simulink model "Biped_Model"  (R2019a)
settings: Solver=VariableStepAuto  StartTime=0.0  StopTime=Time(end)  FixedStep=.001  EnableMultiTasking=on
PreLoadFcn:
  | YBT_HomeDir = pwd;
  | 
  | % Code to use copy within this repository
  | addpath([YBT_HomeDir filesep 'Libraries' filesep 'CFL_Libs']);
  | startup_Contact_Forces
  | 
  | cd(YBT_HomeDir)
  | addpath(YBT_HomeDir);
  | addpath([YBT_HomeDir filesep 'Libraries']);
  | addpath([YBT_HomeDir filesep 'Images']);
  | 
  | Robot_Parameters
model workspace: external: MATLAB File C:\Users\nozaripo\Desktop\BipedalWalking_Simulink_ModelnData\Robot_Parameters.m (data not in the file)
values from neighbouring files (symbols this model uses):
  ankle_servo_kd = 4    [Robot_Parameters.m]
  ankle_servo_ki = 0    [Robot_Parameters.m]
  ankle_servo_kp = 70    [Robot_Parameters.m]
  ankle_to_midLow = 19    [Robot_Parameters.m]
  contact_damping = 50    [Robot_Parameters.m]
  contact_point_radius = 0.005    [Robot_Parameters.m]
  contact_stiffness = 90311    [Robot_Parameters.m]
  deriv_filter_coeff = 50    [Robot_Parameters.m]
  foot_mass = 1    [Robot_Parameters.m]
  height_plane = 0.1    [Robot_Parameters.m]
  hip_servo_kd = 30    [Robot_Parameters.m]
  hip_servo_ki = 0    [Robot_Parameters.m]
  hip_servo_kp = 300    [Robot_Parameters.m]
  init = -joint_angles(1,:)    [Script_Data.m]
  init_vel = -vel(1,:)    [Script_Data.m]
  joint_angles = joint_angles(:,end:-1:1)    [Script_Data.m]
  joint_damping = 0    [Robot_Parameters.m]
  joint_stiffness = 0    [Robot_Parameters.m]
  knee_servo_kd = 30    [Robot_Parameters.m]
  knee_servo_ki = 0    [Robot_Parameters.m]
  knee_servo_kp = 150    [Robot_Parameters.m]
  knee_to_midUpp = 19    [Robot_Parameters.m]
  linear_contact_flag = 0    [Robot_Parameters.m]
  lower_leg_CM_offset = 2.55    [Robot_Parameters.m]
  lower_leg_mass = 2.87    [Robot_Parameters.m]
  max_torque_ank = 45    [Robot_Parameters.m]
  max_torque_hip = 25    [Robot_Parameters.m]
  max_torque_kn = 30    [Robot_Parameters.m]
  midLow_to_knee = 19    [Robot_Parameters.m]
  midUpp_to_hip = 19    [Robot_Parameters.m]
  motion_time_constant = 0.01    [Robot_Parameters.m]
  motor_constant = 0.01    [Robot_Parameters.m]
  motor_inertia = 0    [Robot_Parameters.m]
  mu_k = 0.5    [Robot_Parameters.m]
  mu_s = 0.8    [Robot_Parameters.m]
  mu_vth = 0.1    [Robot_Parameters.m]
  pen_exp = 1.5    [Robot_Parameters.m]
  plane_x = 3    [Robot_Parameters.m]
  plane_y = 0.3    [Robot_Parameters.m]
  split_belt = 0    [Script_Data.m]
  Time = (0:.01:.01*209)'    [Script_Data.m]
  torso_mass = 27.17    [Robot_Parameters.m]
  torso_to_hip = 11    [Robot_Parameters.m]
  upper_leg_CM_offset = 2.55    [Robot_Parameters.m]
  upper_leg_length = 38    [Robot_Parameters.m]
  upper_leg_mass = 4.7    [Robot_Parameters.m]
  V_treadmill = -1.0    (= -1)    [Script_Data.m]
  YBT_Par = struct    [Robot_Parameters.m]
undefined symbols (not defined in the file or in its folder): Extr_Data_LinkHoles, X, Y, Z
libraries: nesl_utility x198, sm_lib x144, fl_lib x42, simulink x20, ee_lib x18, Contact_Forces_Lib x16, Parts_Lib x10, Multibody_Multiphysics_Lib x6, simulink_extras x1
(part 9 of 11)

== system Biped_Model/Robot/Robot Leg R/Package Measurements/Extract Measurements1 ==
  meas : Inport
  Bus Selector : BusSelector  OutputSignals=angle,speed,torque
  angle : Outport
  speed : Outport  Port=2
  torque : Outport  Port=3
  wires:
  Bus Selector/3 -> torque/1  "<torque>"
  meas/1 -> Bus Selector/1
  Bus Selector/1 -> angle/1  "<angle>"
  Bus Selector/2 -> speed/1  "<speed>"

== system Biped_Model/Robot/Robot Leg R/Package Measurements/Extract Measurements2 ==
  meas : Inport
  Bus Selector : BusSelector  OutputSignals=angle,speed,torque
  angle : Outport
  speed : Outport  Port=2
  torque : Outport  Port=3
  wires:
  Bus Selector/1 -> angle/1  "<angle>"
  meas/1 -> Bus Selector/1
  Bus Selector/3 -> torque/1  "<torque>"
  Bus Selector/2 -> speed/1  "<speed>"

== system Biped_Model/Robot/Robot Leg L/Ankle Joint/Motor/Joint Servo ==
  qref : Inport
  Abs : Abs
  Controlled Voltage Source : fl_lib/Electrical/Electrical Sources/Controlled Voltage Source
  Controlled Voltage Source1 : fl_lib/Electrical/Electrical Sources/Controlled Voltage Source
  Electrical Reference : fl_lib/Electrical/Electrical Elements/Electrical Reference
  PID Controller : simulink/Continuous/PID Controller  Controller=PID  Form=Parallel  TimeDomain=Continuous-time  SampleTime=-1  IntegratorMethod=Forward Euler  FilterMethod=Forward Euler  ControllerParametersSource=internal  P=Kp  I=Ki  D=Kd  UseFilter=on  N=N  TunerSelectOption=Transfer Function Based (PID Tuner App)  ZeroCross=off  InitialConditionSource=internal  InitialConditionForIntegrator=0  InitialConditionForFilter=0  DifferentiatorICPrevScaledInput=0  ExternalReset=none  TrackingMode=off  Kt=1  LimitOutput=on  UpperSaturationLimit=Tmax  LowerSaturationLimit=-Tmax  LinearizeAsGain=on  AntiWindupMode=clamping  Kb=1  POutMin=[]  POutMax=[]  IOutMin=[]  IOutMax=[]  DOutMin=[]  DOutMax=[]  NOutMin=[]  NOutMax=[]  SumOutMin=[]  SumOutMax=[]  SaturationOutMin=[]  SaturationOutMax=[]  PParamMin=[]  PParamMax=[]  IParamMin=[]  IParamMax=[]  DParamMin=[]  DParamMax=[]  NParamMin=[]  NParamMax=[]  KbParamMin=[]  KbParamMax=[]  KtParamMin=[]  KtParamMax=[]  KbOutMin=[]  KbOutMax=[]  KtOutMin=[]  KtOutMax=[]  IntegratorOutMin=[]  IntegratorOutMax=[]  FilterOutMin=[]  FilterOutMax=[]  SumI1OutMin=[]  SumI1OutMax=[]  SumI2OutMin=[]  SumI2OutMax=[]  SumI3OutMin=[]  SumI3OutMax=[]  SumI4OutMin=[]  SumI4OutMax=[]  SumDOutMin=[]  SumDOutMax=[]  DifferentiatorOutMin=[]  DifferentiatorOutMax=[]  FilterDiffOutCoefMin=[]  FilterDiffOutCoefMax=[]  ReciprocalOutMin=[]  ReciprocalOutMax=[]  SumDenOutMin=[]  SumDenOutMax=[]  SumNumOutMin=[]  SumNumOutMax=[]  DivideOutMin=[]  DivideOutMax=[]  IntegratorContinuousStateAttributes=''  IntegratorStateMustResolveToSignalObject=off  IntegratorRTWStateStorageClass=Auto  FilterContinuousStateAttributes=''  FilterStateMustResolveToSignalObject=off  FilterRTWStateStorageClass=Auto  ParallelPVariant=InternalParameters  IdealPVariant=Disabled  IVariant=InternalParameters  DVariant=InternalParameters  IntegratorVariant=Continuous  SatVariant=Enabled  AWVariant=ContClampingParallel  PCopyVariant=Disabled  TRVariant=Disabled  FdbkBlocksVariant=Forward  IdealPFdbkVariant=Disabled  SatFdbkVariant=Disabled  DerivativeFilterVariant=ContFilter  NVariant=InternalParameters  NCopyVariant=Disabled  FilterICVariant=InternalICsFilter  IntegratorICVariant=InternalICs  ExternalResetVariant=Disabled  TRSumVariant=Passthrough  SumFdbkVariant=Disabled  SumVariant=Sum_PID
  PS-Simulink Converter : nesl_utility/PS-Simulink Converter  PhysicalDomain=network_engine_domain  SubClassName=ps_output  LeftPortType=input  RightPortType=output  PseudoPeriodic=off  Frequencies=[]  Unit=rad  AffineConversion=off
  Relay : Relay  OnSwitchValue=1e-3  OffSwitchValue=-1e-3  OnOutputValue=0  OffOutputValue=5
  Simulink-PS Converter : nesl_utility/Simulink-PS Converter  PhysicalDomain=network_engine_domain  SubClassName=ps_input  LeftPortType=input  RightPortType=output  PseudoPeriodic=off  Frequencies=[]  NoiseDistribution=none  NoiseParameters=[]  Unit=1  AffineConversion=off  FilteringAndDerivatives=provide  SimscapeFilterOrder=1  InputFilterTimeConstant=0.005  UdotUserProvided=0
  Simulink-PS Converter1 : nesl_utility/Simulink-PS Converter  PhysicalDomain=network_engine_domain  SubClassName=ps_input  LeftPortType=input  RightPortType=output  PseudoPeriodic=off  Frequencies=[]  NoiseDistribution=none  NoiseParameters=[]  Unit=1  AffineConversion=off  FilteringAndDerivatives=provide  SimscapeFilterOrder=1  InputFilterTimeConstant=0.005  UdotUserProvided=0
  Sum : Sum  Inputs=|+-
  q : PMIOPort  Side=Left
  V : PMIOPort  Port=2  Side=Right
  REV : PMIOPort  Port=3  Side=Right
  wires:
  PID Controller/1 -> Abs/1, Relay/1
  qref/1 -> Sum/1
  PS-Simulink Converter/1 -> Sum/2
  Sum/1 -> PID Controller/1
  Abs/1 -> Simulink-PS Converter/1
  Relay/1 -> Simulink-PS Converter1/1
  connections:
  q/RConn1 -- PS-Simulink Converter/LConn1
  Simulink-PS Converter/RConn1 -- Controlled Voltage Source/RConn1
  Controlled Voltage Source/LConn1 -- V/RConn1
  Electrical Reference/LConn1 -- Controlled Voltage Source/RConn2 -- Controlled Voltage Source1/RConn2
  Controlled Voltage Source1/LConn1 -- REV/RConn1
  Simulink-PS Converter1/RConn1 -- Controlled Voltage Source1/RConn1

== system Biped_Model/Robot/Robot Leg L/Ankle Joint/Torque/Joint Servo ==
  qref : Inport
  Memory : Memory
  PID Controller : simulink/Continuous/PID Controller  Controller=PID  Form=Parallel  TimeDomain=Continuous-time  SampleTime=-1  IntegratorMethod=Forward Euler  FilterMethod=Forward Euler  ControllerParametersSource=internal  P=Kp  I=Ki  D=Kd  UseFilter=on  N=N  TunerSelectOption=Transfer Function Based (PID Tuner App)  ZeroCross=off  InitialConditionSource=internal  InitialConditionForIntegrator=0  InitialConditionForFilter=0  DifferentiatorICPrevScaledInput=0  ExternalReset=none  TrackingMode=off  Kt=1  LimitOutput=on  UpperSaturationLimit=Tmax  LowerSaturationLimit=-Tmax  LinearizeAsGain=on  AntiWindupMode=clamping  Kb=1  POutMin=[]  POutMax=[]  IOutMin=[]  IOutMax=[]  DOutMin=[]  DOutMax=[]  NOutMin=[]  NOutMax=[]  SumOutMin=[]  SumOutMax=[]  SaturationOutMin=[]  SaturationOutMax=[]  PParamMin=[]  PParamMax=[]  IParamMin=[]  IParamMax=[]  DParamMin=[]  DParamMax=[]  NParamMin=[]  NParamMax=[]  KbParamMin=[]  KbParamMax=[]  KtParamMin=[]  KtParamMax=[]  KbOutMin=[]  KbOutMax=[]  KtOutMin=[]  KtOutMax=[]  IntegratorOutMin=[]  IntegratorOutMax=[]  FilterOutMin=[]  FilterOutMax=[]  SumI1OutMin=[]  SumI1OutMax=[]  SumI2OutMin=[]  SumI2OutMax=[]  SumI3OutMin=[]  SumI3OutMax=[]  SumI4OutMin=[]  SumI4OutMax=[]  SumDOutMin=[]  SumDOutMax=[]  DifferentiatorOutMin=[]  DifferentiatorOutMax=[]  FilterDiffOutCoefMin=[]  FilterDiffOutCoefMax=[]  ReciprocalOutMin=[]  ReciprocalOutMax=[]  SumDenOutMin=[]  SumDenOutMax=[]  SumNumOutMin=[]  SumNumOutMax=[]  DivideOutMin=[]  DivideOutMax=[]  IntegratorContinuousStateAttributes=''  IntegratorStateMustResolveToSignalObject=off  IntegratorRTWStateStorageClass=Auto  FilterContinuousStateAttributes=''  FilterStateMustResolveToSignalObject=off  FilterRTWStateStorageClass=Auto  ParallelPVariant=InternalParameters  IdealPVariant=Disabled  IVariant=InternalParameters  DVariant=InternalParameters  IntegratorVariant=Continuous  SatVariant=Enabled  AWVariant=ContClampingParallel  PCopyVariant=Disabled  TRVariant=Disabled  FdbkBlocksVariant=Forward  IdealPFdbkVariant=Disabled  SatFdbkVariant=Disabled  DerivativeFilterVariant=ContFilter  NVariant=InternalParameters  NCopyVariant=Disabled  FilterICVariant=InternalICsFilter  IntegratorICVariant=InternalICs  ExternalResetVariant=Disabled  TRSumVariant=Passthrough  SumFdbkVariant=Disabled  SumVariant=Sum_PID
  PS-Simulink Converter : nesl_utility/PS-Simulink Converter  PhysicalDomain=network_engine_domain  SubClassName=ps_output  LeftPortType=input  RightPortType=output  PseudoPeriodic=off  Frequencies=[]  Unit=rad  AffineConversion=off
  Sum : Sum  Inputs=|+-
  q : PMIOPort  Side=Left
  t : Outport
  wires:
  PID Controller/1 -> t/1
  Sum/1 -> PID Controller/1
  PS-Simulink Converter/1 -> Memory/1
  qref/1 -> Sum/1
  Memory/1 -> Sum/2
  connections:
  q/RConn1 -- PS-Simulink Converter/LConn1

== system Biped_Model/Robot/Robot Leg L/Box to Belt In Force1/Sphere to Plane Force Enabled nz1/Check Sphere on Plane ==
  x : Inport
  y : Inport  Port=2
  Abs : Abs  ZeroCross=off
  Abs1 : Abs  ZeroCross=off
  Check loc x-axis : simulink/Logic and Bit Operations/Compare To Constant  relop=<  const=plane_lenx  OutDataTypeStr=boolean  ZeroCross=off
  Check loc y-axis : simulink/Logic and Bit Operations/Compare To Constant  relop=<  const=plane_leny  OutDataTypeStr=boolean  ZeroCross=off
  Data Type Conversion : DataTypeConversion
  Gain : Gain  Gain=2
  Gain1 : Gain  Gain=2
  Logical Operator : Logic  AllPortsSameDT=off  OutDataTypeStr=boolean
  En : Outport
  wires:
  Check loc x-axis/1 -> Logical Operator/1
  Logical Operator/1 -> Data Type Conversion/1
  y/1 -> Gain1/1
  Data Type Conversion/1 -> En/1
  x/1 -> Gain/1
  Gain/1 -> Abs/1
  Gain1/1 -> Abs1/1
  Abs/1 -> Check loc x-axis/1
  Abs1/1 -> Check loc y-axis/1
  Check loc y-axis/1 -> Logical Operator/2

== system Biped_Model/Robot/Robot Leg L/Box to Belt In Force1/Sphere to Plane Force Enabled nz1/Demux ==
  Frc : Inport
  Demux : Demux
  Simulink-PS Converter{,1..2,6} (4 alike) : nesl_utility/Simulink-PS Converter  PhysicalDomain=network_engine_domain  SubClassName=ps_input  LeftPortType=input  RightPortType=output  PseudoPeriodic=off  Frequencies=[]  NoiseDistribution=none  NoiseParameters=[]  Unit=1  AffineConversion=off  FilteringAndDerivatives=zero  SimscapeFilterOrder=1  InputFilterTimeConstant=0.001  UdotUserProvided=1
  FSph : PMIOPort  Side=Right
  TSph : PMIOPort  Port=2  Side=Right
  FPla : PMIOPort  Port=3  Side=Right
  TPla : PMIOPort  Port=4  Side=Right
  wires:
  Demux/3 -> Simulink-PS Converter6/1
  Demux/4 -> Simulink-PS Converter2/1
  Demux/2 -> Simulink-PS Converter1/1
  Demux/1 -> Simulink-PS Converter/1
  Frc/1 -> Demux/1
  connections:
  Simulink-PS Converter6/RConn1 -- FPla/RConn1
  Simulink-PS Converter1/RConn1 -- TSph/RConn1
  Simulink-PS Converter/RConn1 -- FSph/RConn1
  Simulink-PS Converter2/RConn1 -- TPla/RConn1

== system Biped_Model/Robot/Robot Leg L/Box to Belt In Force1/Sphere to Plane Force Enabled nz1/Enable Outputs ==
  Frc : Inport
  En : Inport  Port=2
  FrameSep : Inport  Port=3
  Bus Creator1 : BusCreator  Inputs=7
  Bus Selector : BusSelector  OutputSignals=Normal Force,Friction Force,Penetration,Penetration Vel,Spr Force,Damp Force
  Demux : Demux  Outputs=[1 3 1 1 1 1]
  Mux : Mux  Inputs=6
  Product : Product
  Out : Outport
  wires:
  Bus Selector/5 -> Mux/5  "<Spr Force>"
  Bus Selector/6 -> Mux/6  "<Damp Force>"
  Bus Selector/1 -> Mux/1  "<Normal Force>"
  FrameSep/1 -> Bus Creator1/7
  Bus Selector/4 -> Mux/4  "<Penetration Vel>"
  Frc/1 -> Bus Selector/1
  Bus Selector/2 -> Mux/2  "<Friction Force>"
  Bus Creator1/1 -> Out/1
  Bus Selector/3 -> Mux/3  "<Penetration>"
  Mux/1 -> Product/2
  En/1 -> Product/1
  Product/1 -> Demux/1
  Demux/3 -> Bus Creator1/3  "Penetration"
  Demux/5 -> Bus Creator1/5  "Spr Force"
  Demux/4 -> Bus Creator1/4  "Penetration Vel"
  Demux/6 -> Bus Creator1/6  "Damp Force"
  Demux/1 -> Bus Creator1/1  "Normal Force"
  Demux/2 -> Bus Creator1/2  "Friction Force"

== system Biped_Model/Robot/Robot Leg L/Box to Belt In Force1/Sphere to Plane Force Enabled nz1/Forces ==
  x : Inport
  y : Inport  Port=2
  z : Inport  Port=3
  vz : Inport  Port=4
  R : Inport  Port=5
  wx : Inport  Port=6
  wy : Inport  Port=7
  vx : Inport  Port=8
  vy : Inport  Port=9
  Action Port : ActionPort  ActionPortLabel=if((u1 > 0 & u2>0))
  Bus Creator : BusCreator  Inputs=6
  Calculate Penetration : Subsystem
  Copy for Merge : SignalConversion  OverrideOpt=off
  Cross Product : Contact_Forces_Lib/Math/Cross Product  SystemSampleTime=-1
      settings: SourceProductName=Simscape Multibody Contact Forces Library
  Ff : Subsystem
  Fn : Subsystem
  Force Law : Subsystem  AncestorBlock=Contact_Forces_Lib/Force Law  VariantControlMode=Label  Variant=on  LabelModeActiveChoice=Linear
  Mux : Mux
  Mux2 : Mux  Inputs=3
  Product : Product
  Product1 : Product
  Sum : Sum
  Sum1 : Sum
  z1 : InportShadow  Port=3
  Frc : Outport
  Out : Outport  Port=2
  wires:
  Cross Product/1 -> Mux/4  "TPla"
  Ff/2(T Sph) -> Mux/2  "TSph"
  Sum/1 -> Mux/1  "FSph"
  wx/1 -> Ff/4(wx)
  wy/1 -> Ff/5(wy)
  vy/1 -> Ff/7(vy)
  Ff/3(Ff Pla) -> Bus Creator/6, Sum1/2  "Friction Force"
  x/1 -> Mux2/1
  z/1 -> Mux2/3
  y/1 -> Mux2/2
  Fn/1(Fn) -> Bus Creator/5  "Normal Force"
  Ff/1(Ff Sph) -> Sum/2
  Mux2/1 -> Cross Product/1
  Sum1/1 -> Cross Product/2, Copy for Merge/1  "FPla"
  Force Law/2(Damp F) -> Product1/1
  R/1 -> Ff/2(R), Fn/1(R)
  Calculate Penetration/4(Vel Sign) -> Product1/2
  Calculate Penetration/1(Pos Sign) -> Product/1, Ff/3(zSign)
  Fn/3(FnB) -> Ff/1(Fn), Sum1/1
  Calculate Penetration/3(Pen Vel) -> Force Law/2(Pen Vel), Bus Creator/2  "Penetration Vel"
  Calculate Penetration/2(Pen) -> Force Law/1(Pen), Bus Creator/1  "Penetration"
  z1/1 -> Calculate Penetration/1(z)
  vz/1 -> Calculate Penetration/2(vz)
  Force Law/1(Spr F) -> Product/2
  Bus Creator/1 -> Out/1
  Mux/1 -> Frc/1
  Fn/2(FnF) -> Sum/1
  Product/1 -> Fn/2(SprF), Bus Creator/3  "Spr Force"
  Product1/1 -> Fn/3(DamF), Bus Creator/4  "Damp Force"
  vx/1 -> Ff/6(vx)
  Copy for Merge/1 -> Mux/3

== system Biped_Model/Robot/Robot Leg L/Box to Belt In Force1/Sphere to Plane Force Enabled nz1/No Force ==
  Action Port : ActionPort  ActionPortLabel=else
  Zeros : Constant  Value=[0 0 0 0 0 0 0 0 0 0 0 0]  SampleTime=0
  Frc : Outport  InitialOutput=[0 0 0 0 0 0 0 0 0 0 0 0]
  wires:
  Zeros/1 -> Frc/1

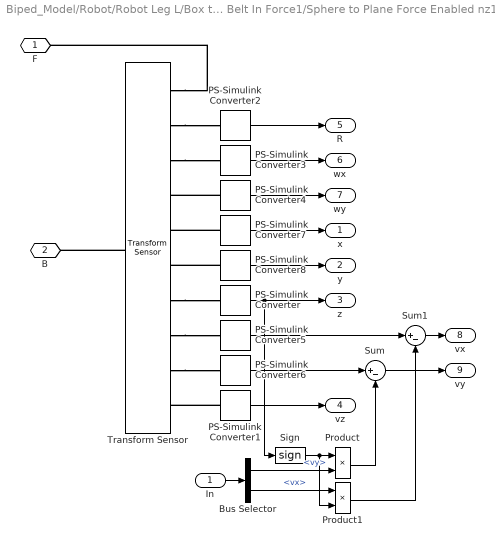
== system Biped_Model/Robot/Robot Leg L/Box to Belt In Force1/Sphere to Plane Force Enabled nz1/Sensing ==
  In : Inport
  Bus Selector : BusSelector  OutputSignals=vy,vx
  PS-Simulink Converter : nesl_utility/PS-Simulink Converter  PhysicalDomain=network_engine_domain  SubClassName=ps_output  LeftPortType=input  RightPortType=output  PseudoPeriodic=off  Frequencies=[]  Unit=m  AffineConversion=off
  PS-Simulink Converter1 : nesl_utility/PS-Simulink Converter  PhysicalDomain=network_engine_domain  SubClassName=ps_output  LeftPortType=input  RightPortType=output  PseudoPeriodic=off  Frequencies=[]  Unit=m/s  AffineConversion=off
  PS-Simulink Converter2 : nesl_utility/PS-Simulink Converter  PhysicalDomain=network_engine_domain  SubClassName=ps_output  LeftPortType=input  RightPortType=output  PseudoPeriodic=off  Frequencies=[]  Unit=1  AffineConversion=off
  PS-Simulink Converter3 : nesl_utility/PS-Simulink Converter  PhysicalDomain=network_engine_domain  SubClassName=ps_output  LeftPortType=input  RightPortType=output  PseudoPeriodic=off  Frequencies=[]  Unit=1  AffineConversion=off
  PS-Simulink Converter4 : nesl_utility/PS-Simulink Converter  PhysicalDomain=network_engine_domain  SubClassName=ps_output  LeftPortType=input  RightPortType=output  PseudoPeriodic=off  Frequencies=[]  Unit=1  AffineConversion=off
  PS-Simulink Converter5 : nesl_utility/PS-Simulink Converter  PhysicalDomain=network_engine_domain  SubClassName=ps_output  LeftPortType=input  RightPortType=output  PseudoPeriodic=off  Frequencies=[]  Unit=m/s  AffineConversion=off
  PS-Simulink Converter6 : nesl_utility/PS-Simulink Converter  PhysicalDomain=network_engine_domain  SubClassName=ps_output  LeftPortType=input  RightPortType=output  PseudoPeriodic=off  Frequencies=[]  Unit=m/s  AffineConversion=off
  PS-Simulink Converter7 : nesl_utility/PS-Simulink Converter  PhysicalDomain=network_engine_domain  SubClassName=ps_output  LeftPortType=input  RightPortType=output  PseudoPeriodic=off  Frequencies=[]  Unit=m  AffineConversion=off
  PS-Simulink Converter8 : nesl_utility/PS-Simulink Converter  PhysicalDomain=network_engine_domain  SubClassName=ps_output  LeftPortType=input  RightPortType=output  PseudoPeriodic=off  Frequencies=[]  Unit=m  AffineConversion=off
  Product : Product
  Product1 : Product
  Sign : Signum  ZeroCross=off
  Sum : Sum  Inputs=|+-
  Sum1 : Sum  Inputs=|+-
  Transform Sensor : sm_lib/Frames and Transforms/Transform Sensor  MeasurementFrame=Base  SenseAngle=off  SenseAxis=off  SenseAngle1=off  SenseAngle2=off  SenseAngle3=off  SenseQ=off  SenseR=on  SenseOmegaX=on  SenseOmegaY=on  SenseOmegaZ=off  SenseOmega1=off  SenseOmega2=off  SenseOmega3=off  SenseQDot=off  SenseRDot=off  SenseAlphaX=off  SenseAlphaY=off  SenseAlphaZ=off  SenseAlpha1=off  SenseAlpha2=off  SenseAlpha3=off  SenseQDDot=off  SenseRDDot=off  SenseX=on  SenseY=on  SenseZ=on  SenseRad=off  SenseAzim=off  SenseDist=off  SenseInc=off  SenseXDot=on  SenseYDot=on  SenseZDot=on  SenseRadDot=off  SenseAzimDot=off  SenseDistDot=off  SenseIncDot=off  SenseXDDot=off  SenseYDDot=off  SenseZDDot=off  SenseRadDDot=off  SenseAzimDDot=off  SenseDistDDot=off  SenseIncDDot=off
  F : PMIOPort  Side=Left
  B : PMIOPort  Port=2  Side=Left
  x : Outport
  y : Outport  Port=2
  z : Outport  Port=3
  vz : Outport  Port=4
  R : Outport  Port=5
  wx : Outport  Port=6
  wy : Outport  Port=7
  vx : Outport  Port=8
  vy : Outport  Port=9
  wires:
  Bus Selector/2 -> Product1/1  "<vx>"
  Product1/1 -> Sum1/2
  Sum1/1 -> vx/1
  Sum/1 -> vy/1
  PS-Simulink Converter6/1 -> Sum/1
  Product/1 -> Sum/2
  Sign/1 -> Product/1, Product1/2
  Bus Selector/1 -> Product/2  "<vy>"
  In/1 -> Bus Selector/1
  PS-Simulink Converter5/1 -> Sum1/1
  PS-Simulink Converter8/1 -> y/1
  PS-Simulink Converter7/1 -> x/1
  PS-Simulink Converter4/1 -> wy/1
  PS-Simulink Converter3/1 -> wx/1
  PS-Simulink Converter2/1 -> R/1
  PS-Simulink Converter/1 -> z/1, Sign/1
  PS-Simulink Converter1/1 -> vz/1
  connections:
  PS-Simulink Converter8/LConn1 -- Transform Sensor/RConn6
  PS-Simulink Converter7/LConn1 -- Transform Sensor/RConn5
  Transform Sensor/RConn7 -- PS-Simulink Converter/LConn1
  Transform Sensor/RConn8 -- PS-Simulink Converter5/LConn1
  Transform Sensor/RConn9 -- PS-Simulink Converter6/LConn1
  PS-Simulink Converter1/LConn1 -- Transform Sensor/RConn10
  PS-Simulink Converter4/LConn1 -- Transform Sensor/RConn4
  Transform Sensor/RConn3 -- PS-Simulink Converter3/LConn1
  Transform Sensor/RConn2 -- PS-Simulink Converter2/LConn1
  Transform Sensor/LConn1 -- B/RConn1
  Transform Sensor/RConn1 -- F/RConn1

== system Biped_Model/Robot/Robot Leg L/Box to Belt In Force1/Sphere to Plane Force Enabled nz2/Check Sphere on Plane ==
  x : Inport
  y : Inport  Port=2
  Abs : Abs  ZeroCross=off
  Abs1 : Abs  ZeroCross=off
  Check loc x-axis : simulink/Logic and Bit Operations/Compare To Constant  relop=<  const=plane_lenx  OutDataTypeStr=boolean  ZeroCross=off
  Check loc y-axis : simulink/Logic and Bit Operations/Compare To Constant  relop=<  const=plane_leny  OutDataTypeStr=boolean  ZeroCross=off
  Data Type Conversion : DataTypeConversion
  Gain : Gain  Gain=2
  Gain1 : Gain  Gain=2
  Logical Operator : Logic  AllPortsSameDT=off  OutDataTypeStr=boolean
  En : Outport
  wires:
  Check loc y-axis/1 -> Logical Operator/2
  Abs1/1 -> Check loc y-axis/1
  Abs/1 -> Check loc x-axis/1
  Gain1/1 -> Abs1/1
  Gain/1 -> Abs/1
  x/1 -> Gain/1
  Data Type Conversion/1 -> En/1
  y/1 -> Gain1/1
  Logical Operator/1 -> Data Type Conversion/1
  Check loc x-axis/1 -> Logical Operator/1

== system Biped_Model/Robot/Robot Leg L/Box to Belt In Force1/Sphere to Plane Force Enabled nz2/Demux ==
  Frc : Inport
  Demux : Demux
  Simulink-PS Converter{,1..2,6} (4 alike) : nesl_utility/Simulink-PS Converter  PhysicalDomain=network_engine_domain  SubClassName=ps_input  LeftPortType=input  RightPortType=output  PseudoPeriodic=off  Frequencies=[]  NoiseDistribution=none  NoiseParameters=[]  Unit=1  AffineConversion=off  FilteringAndDerivatives=zero  SimscapeFilterOrder=1  InputFilterTimeConstant=0.001  UdotUserProvided=1
  FSph : PMIOPort  Side=Right
  TSph : PMIOPort  Port=2  Side=Right
  FPla : PMIOPort  Port=3  Side=Right
  TPla : PMIOPort  Port=4  Side=Right
  wires:
  Frc/1 -> Demux/1
  Demux/1 -> Simulink-PS Converter/1
  Demux/2 -> Simulink-PS Converter1/1
  Demux/4 -> Simulink-PS Converter2/1
  Demux/3 -> Simulink-PS Converter6/1
  connections:
  Simulink-PS Converter2/RConn1 -- TPla/RConn1
  Simulink-PS Converter/RConn1 -- FSph/RConn1
  Simulink-PS Converter1/RConn1 -- TSph/RConn1
  Simulink-PS Converter6/RConn1 -- FPla/RConn1

== system Biped_Model/Robot/Robot Leg L/Box to Belt In Force1/Sphere to Plane Force Enabled nz2/Enable Outputs ==
  Frc : Inport
  En : Inport  Port=2
  FrameSep : Inport  Port=3
  Bus Creator1 : BusCreator  Inputs=7
  Bus Selector : BusSelector  OutputSignals=Normal Force,Friction Force,Penetration,Penetration Vel,Spr Force,Damp Force
  Demux : Demux  Outputs=[1 3 1 1 1 1]
  Mux : Mux  Inputs=6
  Product : Product
  Out : Outport
  wires:
  Demux/2 -> Bus Creator1/2  "Friction Force"
  Demux/1 -> Bus Creator1/1  "Normal Force"
  Demux/6 -> Bus Creator1/6  "Damp Force"
  Demux/4 -> Bus Creator1/4  "Penetration Vel"
  Demux/5 -> Bus Creator1/5  "Spr Force"
  Demux/3 -> Bus Creator1/3  "Penetration"
  Product/1 -> Demux/1
  En/1 -> Product/1
  Mux/1 -> Product/2
  Bus Selector/3 -> Mux/3  "<Penetration>"
  Bus Creator1/1 -> Out/1
  Bus Selector/2 -> Mux/2  "<Friction Force>"
  Frc/1 -> Bus Selector/1
  Bus Selector/4 -> Mux/4  "<Penetration Vel>"
  FrameSep/1 -> Bus Creator1/7
  Bus Selector/1 -> Mux/1  "<Normal Force>"
  Bus Selector/6 -> Mux/6  "<Damp Force>"
  Bus Selector/5 -> Mux/5  "<Spr Force>"

== system Biped_Model/Robot/Robot Leg L/Box to Belt In Force1/Sphere to Plane Force Enabled nz2/Forces ==
  x : Inport
  y : Inport  Port=2
  z : Inport  Port=3
  vz : Inport  Port=4
  R : Inport  Port=5
  wx : Inport  Port=6
  wy : Inport  Port=7
  vx : Inport  Port=8
  vy : Inport  Port=9
  Action Port : ActionPort  ActionPortLabel=if((u1 > 0 & u2>0))
  Bus Creator : BusCreator  Inputs=6
  Calculate Penetration : Subsystem
  Copy for Merge : SignalConversion  OverrideOpt=off
  Cross Product : Contact_Forces_Lib/Math/Cross Product  SystemSampleTime=-1
      settings: SourceProductName=Simscape Multibody Contact Forces Library
  Ff : Subsystem
  Fn : Subsystem
  Force Law : Subsystem  AncestorBlock=Contact_Forces_Lib/Force Law  VariantControlMode=Label  Variant=on  LabelModeActiveChoice=Linear
  Mux : Mux
  Mux2 : Mux  Inputs=3
  Product : Product
  Product1 : Product
  Sum : Sum
  Sum1 : Sum
  z1 : InportShadow  Port=3
  Frc : Outport
  Out : Outport  Port=2
  wires:
  Copy for Merge/1 -> Mux/3
  vx/1 -> Ff/6(vx)
  Product1/1 -> Bus Creator/4, Fn/3(DamF)  "Damp Force"
  Product/1 -> Bus Creator/3, Fn/2(SprF)  "Spr Force"
  Fn/2(FnF) -> Sum/1
  Mux/1 -> Frc/1
  Bus Creator/1 -> Out/1
  Force Law/1(Spr F) -> Product/2
  vz/1 -> Calculate Penetration/2(vz)
  z1/1 -> Calculate Penetration/1(z)
  Calculate Penetration/2(Pen) -> Bus Creator/1, Force Law/1(Pen)  "Penetration"
  Calculate Penetration/3(Pen Vel) -> Bus Creator/2, Force Law/2(Pen Vel)  "Penetration Vel"
  Fn/3(FnB) -> Sum1/1, Ff/1(Fn)
  Calculate Penetration/1(Pos Sign) -> Ff/3(zSign), Product/1
  Calculate Penetration/4(Vel Sign) -> Product1/2
  R/1 -> Fn/1(R), Ff/2(R)
  Force Law/2(Damp F) -> Product1/1
  Sum1/1 -> Copy for Merge/1, Cross Product/2  "FPla"
  Mux2/1 -> Cross Product/1
  Ff/1(Ff Sph) -> Sum/2
  Fn/1(Fn) -> Bus Creator/5  "Normal Force"
  y/1 -> Mux2/2
  z/1 -> Mux2/3
  x/1 -> Mux2/1
  Ff/3(Ff Pla) -> Sum1/2, Bus Creator/6  "Friction Force"
  vy/1 -> Ff/7(vy)
  wy/1 -> Ff/5(wy)
  wx/1 -> Ff/4(wx)
  Sum/1 -> Mux/1  "FSph"
  Ff/2(T Sph) -> Mux/2  "TSph"
  Cross Product/1 -> Mux/4  "TPla"

== system Biped_Model/Robot/Robot Leg L/Box to Belt In Force1/Sphere to Plane Force Enabled nz2/No Force ==
  Action Port : ActionPort  ActionPortLabel=else
  Zeros : Constant  Value=[0 0 0 0 0 0 0 0 0 0 0 0]  SampleTime=0
  Frc : Outport  InitialOutput=[0 0 0 0 0 0 0 0 0 0 0 0]
  wires:
  Zeros/1 -> Frc/1

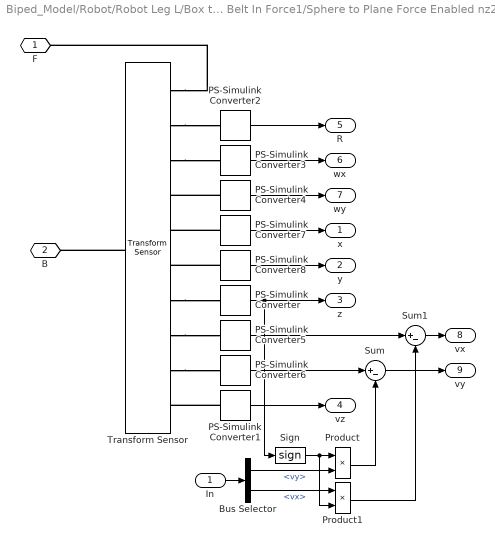
== system Biped_Model/Robot/Robot Leg L/Box to Belt In Force1/Sphere to Plane Force Enabled nz2/Sensing ==
  In : Inport
  Bus Selector : BusSelector  OutputSignals=vy,vx
  PS-Simulink Converter : nesl_utility/PS-Simulink Converter  PhysicalDomain=network_engine_domain  SubClassName=ps_output  LeftPortType=input  RightPortType=output  PseudoPeriodic=off  Frequencies=[]  Unit=m  AffineConversion=off
  PS-Simulink Converter1 : nesl_utility/PS-Simulink Converter  PhysicalDomain=network_engine_domain  SubClassName=ps_output  LeftPortType=input  RightPortType=output  PseudoPeriodic=off  Frequencies=[]  Unit=m/s  AffineConversion=off
  PS-Simulink Converter2 : nesl_utility/PS-Simulink Converter  PhysicalDomain=network_engine_domain  SubClassName=ps_output  LeftPortType=input  RightPortType=output  PseudoPeriodic=off  Frequencies=[]  Unit=1  AffineConversion=off
  PS-Simulink Converter3 : nesl_utility/PS-Simulink Converter  PhysicalDomain=network_engine_domain  SubClassName=ps_output  LeftPortType=input  RightPortType=output  PseudoPeriodic=off  Frequencies=[]  Unit=1  AffineConversion=off
  PS-Simulink Converter4 : nesl_utility/PS-Simulink Converter  PhysicalDomain=network_engine_domain  SubClassName=ps_output  LeftPortType=input  RightPortType=output  PseudoPeriodic=off  Frequencies=[]  Unit=1  AffineConversion=off
  PS-Simulink Converter5 : nesl_utility/PS-Simulink Converter  PhysicalDomain=network_engine_domain  SubClassName=ps_output  LeftPortType=input  RightPortType=output  PseudoPeriodic=off  Frequencies=[]  Unit=m/s  AffineConversion=off
  PS-Simulink Converter6 : nesl_utility/PS-Simulink Converter  PhysicalDomain=network_engine_domain  SubClassName=ps_output  LeftPortType=input  RightPortType=output  PseudoPeriodic=off  Frequencies=[]  Unit=m/s  AffineConversion=off
  PS-Simulink Converter7 : nesl_utility/PS-Simulink Converter  PhysicalDomain=network_engine_domain  SubClassName=ps_output  LeftPortType=input  RightPortType=output  PseudoPeriodic=off  Frequencies=[]  Unit=m  AffineConversion=off
  PS-Simulink Converter8 : nesl_utility/PS-Simulink Converter  PhysicalDomain=network_engine_domain  SubClassName=ps_output  LeftPortType=input  RightPortType=output  PseudoPeriodic=off  Frequencies=[]  Unit=m  AffineConversion=off
  Product : Product
  Product1 : Product
  Sign : Signum  ZeroCross=off
  Sum : Sum  Inputs=|+-
  Sum1 : Sum  Inputs=|+-
  Transform Sensor : sm_lib/Frames and Transforms/Transform Sensor  MeasurementFrame=Base  SenseAngle=off  SenseAxis=off  SenseAngle1=off  SenseAngle2=off  SenseAngle3=off  SenseQ=off  SenseR=on  SenseOmegaX=on  SenseOmegaY=on  SenseOmegaZ=off  SenseOmega1=off  SenseOmega2=off  SenseOmega3=off  SenseQDot=off  SenseRDot=off  SenseAlphaX=off  SenseAlphaY=off  SenseAlphaZ=off  SenseAlpha1=off  SenseAlpha2=off  SenseAlpha3=off  SenseQDDot=off  SenseRDDot=off  SenseX=on  SenseY=on  SenseZ=on  SenseRad=off  SenseAzim=off  SenseDist=off  SenseInc=off  SenseXDot=on  SenseYDot=on  SenseZDot=on  SenseRadDot=off  SenseAzimDot=off  SenseDistDot=off  SenseIncDot=off  SenseXDDot=off  SenseYDDot=off  SenseZDDot=off  SenseRadDDot=off  SenseAzimDDot=off  SenseDistDDot=off  SenseIncDDot=off
  F : PMIOPort  Side=Left
  B : PMIOPort  Port=2  Side=Left
  x : Outport
  y : Outport  Port=2
  z : Outport  Port=3
  vz : Outport  Port=4
  R : Outport  Port=5
  wx : Outport  Port=6
  wy : Outport  Port=7
  vx : Outport  Port=8
  vy : Outport  Port=9
  wires:
  PS-Simulink Converter1/1 -> vz/1
  PS-Simulink Converter/1 -> Sign/1, z/1
  PS-Simulink Converter2/1 -> R/1
  PS-Simulink Converter3/1 -> wx/1
  PS-Simulink Converter4/1 -> wy/1
  PS-Simulink Converter7/1 -> x/1
  PS-Simulink Converter8/1 -> y/1
  PS-Simulink Converter5/1 -> Sum1/1
  In/1 -> Bus Selector/1
  Bus Selector/1 -> Product/2  "<vy>"
  Sign/1 -> Product1/2, Product/1
  Product/1 -> Sum/2
  PS-Simulink Converter6/1 -> Sum/1
  Sum/1 -> vy/1
  Sum1/1 -> vx/1
  Product1/1 -> Sum1/2
  Bus Selector/2 -> Product1/1  "<vx>"
  connections:
  Transform Sensor/RConn1 -- F/RConn1
  Transform Sensor/LConn1 -- B/RConn1
  Transform Sensor/RConn2 -- PS-Simulink Converter2/LConn1
  Transform Sensor/RConn3 -- PS-Simulink Converter3/LConn1
  PS-Simulink Converter4/LConn1 -- Transform Sensor/RConn4
  PS-Simulink Converter1/LConn1 -- Transform Sensor/RConn10
  Transform Sensor/RConn9 -- PS-Simulink Converter6/LConn1
  Transform Sensor/RConn8 -- PS-Simulink Converter5/LConn1
  Transform Sensor/RConn7 -- PS-Simulink Converter/LConn1
  PS-Simulink Converter7/LConn1 -- Transform Sensor/RConn5
  PS-Simulink Converter8/LConn1 -- Transform Sensor/RConn6

== system Biped_Model/Robot/Robot Leg L/Hip Joint/Motor/Joint Servo ==
  qref : Inport
  Abs : Abs
  Controlled Voltage Source : fl_lib/Electrical/Electrical Sources/Controlled Voltage Source
  Controlled Voltage Source1 : fl_lib/Electrical/Electrical Sources/Controlled Voltage Source
  Electrical Reference : fl_lib/Electrical/Electrical Elements/Electrical Reference
  PID Controller : simulink/Continuous/PID Controller  Controller=PID  Form=Parallel  TimeDomain=Continuous-time  SampleTime=-1  IntegratorMethod=Forward Euler  FilterMethod=Forward Euler  ControllerParametersSource=internal  P=Kp  I=Ki  D=Kd  UseFilter=on  N=N  TunerSelectOption=Transfer Function Based (PID Tuner App)  ZeroCross=off  InitialConditionSource=internal  InitialConditionForIntegrator=0  InitialConditionForFilter=0  DifferentiatorICPrevScaledInput=0  ExternalReset=none  TrackingMode=off  Kt=1  LimitOutput=on  UpperSaturationLimit=Tmax  LowerSaturationLimit=-Tmax  LinearizeAsGain=on  AntiWindupMode=clamping  Kb=1  POutMin=[]  POutMax=[]  IOutMin=[]  IOutMax=[]  DOutMin=[]  DOutMax=[]  NOutMin=[]  NOutMax=[]  SumOutMin=[]  SumOutMax=[]  SaturationOutMin=[]  SaturationOutMax=[]  PParamMin=[]  PParamMax=[]  IParamMin=[]  IParamMax=[]  DParamMin=[]  DParamMax=[]  NParamMin=[]  NParamMax=[]  KbParamMin=[]  KbParamMax=[]  KtParamMin=[]  KtParamMax=[]  KbOutMin=[]  KbOutMax=[]  KtOutMin=[]  KtOutMax=[]  IntegratorOutMin=[]  IntegratorOutMax=[]  FilterOutMin=[]  FilterOutMax=[]  SumI1OutMin=[]  SumI1OutMax=[]  SumI2OutMin=[]  SumI2OutMax=[]  SumI3OutMin=[]  SumI3OutMax=[]  SumI4OutMin=[]  SumI4OutMax=[]  SumDOutMin=[]  SumDOutMax=[]  DifferentiatorOutMin=[]  DifferentiatorOutMax=[]  FilterDiffOutCoefMin=[]  FilterDiffOutCoefMax=[]  ReciprocalOutMin=[]  ReciprocalOutMax=[]  SumDenOutMin=[]  SumDenOutMax=[]  SumNumOutMin=[]  SumNumOutMax=[]  DivideOutMin=[]  DivideOutMax=[]  IntegratorContinuousStateAttributes=''  IntegratorStateMustResolveToSignalObject=off  IntegratorRTWStateStorageClass=Auto  FilterContinuousStateAttributes=''  FilterStateMustResolveToSignalObject=off  FilterRTWStateStorageClass=Auto  ParallelPVariant=InternalParameters  IdealPVariant=Disabled  IVariant=InternalParameters  DVariant=InternalParameters  IntegratorVariant=Continuous  SatVariant=Enabled  AWVariant=ContClampingParallel  PCopyVariant=Disabled  TRVariant=Disabled  FdbkBlocksVariant=Forward  IdealPFdbkVariant=Disabled  SatFdbkVariant=Disabled  DerivativeFilterVariant=ContFilter  NVariant=InternalParameters  NCopyVariant=Disabled  FilterICVariant=InternalICsFilter  IntegratorICVariant=InternalICs  ExternalResetVariant=Disabled  TRSumVariant=Passthrough  SumFdbkVariant=Disabled  SumVariant=Sum_PID
  PS-Simulink Converter : nesl_utility/PS-Simulink Converter  PhysicalDomain=network_engine_domain  SubClassName=ps_output  LeftPortType=input  RightPortType=output  PseudoPeriodic=off  Frequencies=[]  Unit=rad  AffineConversion=off
  Relay : Relay  OnSwitchValue=1e-3  OffSwitchValue=-1e-3  OnOutputValue=0  OffOutputValue=5
  Simulink-PS Converter : nesl_utility/Simulink-PS Converter  PhysicalDomain=network_engine_domain  SubClassName=ps_input  LeftPortType=input  RightPortType=output  PseudoPeriodic=off  Frequencies=[]  NoiseDistribution=none  NoiseParameters=[]  Unit=1  AffineConversion=off  FilteringAndDerivatives=provide  SimscapeFilterOrder=1  InputFilterTimeConstant=0.005  UdotUserProvided=0
  Simulink-PS Converter1 : nesl_utility/Simulink-PS Converter  PhysicalDomain=network_engine_domain  SubClassName=ps_input  LeftPortType=input  RightPortType=output  PseudoPeriodic=off  Frequencies=[]  NoiseDistribution=none  NoiseParameters=[]  Unit=1  AffineConversion=off  FilteringAndDerivatives=provide  SimscapeFilterOrder=1  InputFilterTimeConstant=0.005  UdotUserProvided=0
  Sum : Sum  Inputs=|+-
  q : PMIOPort  Side=Left
  V : PMIOPort  Port=2  Side=Right
  REV : PMIOPort  Port=3  Side=Right
  wires:
  PID Controller/1 -> Abs/1, Relay/1
  qref/1 -> Sum/1
  PS-Simulink Converter/1 -> Sum/2
  Sum/1 -> PID Controller/1
  Abs/1 -> Simulink-PS Converter/1
  Relay/1 -> Simulink-PS Converter1/1
  connections:
  q/RConn1 -- PS-Simulink Converter/LConn1
  Simulink-PS Converter/RConn1 -- Controlled Voltage Source/RConn1
  Controlled Voltage Source/LConn1 -- V/RConn1
  Electrical Reference/LConn1 -- Controlled Voltage Source/RConn2 -- Controlled Voltage Source1/RConn2
  Controlled Voltage Source1/LConn1 -- REV/RConn1
  Simulink-PS Converter1/RConn1 -- Controlled Voltage Source1/RConn1

== system Biped_Model/Robot/Robot Leg L/Hip Joint/Torque/Joint Servo ==
  qref : Inport
  Memory : Memory
  PID Controller : simulink/Continuous/PID Controller  Controller=PID  Form=Parallel  TimeDomain=Continuous-time  SampleTime=-1  IntegratorMethod=Forward Euler  FilterMethod=Forward Euler  ControllerParametersSource=internal  P=Kp  I=Ki  D=Kd  UseFilter=on  N=N  TunerSelectOption=Transfer Function Based (PID Tuner App)  ZeroCross=off  InitialConditionSource=internal  InitialConditionForIntegrator=0  InitialConditionForFilter=0  DifferentiatorICPrevScaledInput=0  ExternalReset=none  TrackingMode=off  Kt=1  LimitOutput=on  UpperSaturationLimit=Tmax  LowerSaturationLimit=-Tmax  LinearizeAsGain=on  AntiWindupMode=clamping  Kb=1  POutMin=[]  POutMax=[]  IOutMin=[]  IOutMax=[]  DOutMin=[]  DOutMax=[]  NOutMin=[]  NOutMax=[]  SumOutMin=[]  SumOutMax=[]  SaturationOutMin=[]  SaturationOutMax=[]  PParamMin=[]  PParamMax=[]  IParamMin=[]  IParamMax=[]  DParamMin=[]  DParamMax=[]  NParamMin=[]  NParamMax=[]  KbParamMin=[]  KbParamMax=[]  KtParamMin=[]  KtParamMax=[]  KbOutMin=[]  KbOutMax=[]  KtOutMin=[]  KtOutMax=[]  IntegratorOutMin=[]  IntegratorOutMax=[]  FilterOutMin=[]  FilterOutMax=[]  SumI1OutMin=[]  SumI1OutMax=[]  SumI2OutMin=[]  SumI2OutMax=[]  SumI3OutMin=[]  SumI3OutMax=[]  SumI4OutMin=[]  SumI4OutMax=[]  SumDOutMin=[]  SumDOutMax=[]  DifferentiatorOutMin=[]  DifferentiatorOutMax=[]  FilterDiffOutCoefMin=[]  FilterDiffOutCoefMax=[]  ReciprocalOutMin=[]  ReciprocalOutMax=[]  SumDenOutMin=[]  SumDenOutMax=[]  SumNumOutMin=[]  SumNumOutMax=[]  DivideOutMin=[]  DivideOutMax=[]  IntegratorContinuousStateAttributes=''  IntegratorStateMustResolveToSignalObject=off  IntegratorRTWStateStorageClass=Auto  FilterContinuousStateAttributes=''  FilterStateMustResolveToSignalObject=off  FilterRTWStateStorageClass=Auto  ParallelPVariant=InternalParameters  IdealPVariant=Disabled  IVariant=InternalParameters  DVariant=InternalParameters  IntegratorVariant=Continuous  SatVariant=Enabled  AWVariant=ContClampingParallel  PCopyVariant=Disabled  TRVariant=Disabled  FdbkBlocksVariant=Forward  IdealPFdbkVariant=Disabled  SatFdbkVariant=Disabled  DerivativeFilterVariant=ContFilter  NVariant=InternalParameters  NCopyVariant=Disabled  FilterICVariant=InternalICsFilter  IntegratorICVariant=InternalICs  ExternalResetVariant=Disabled  TRSumVariant=Passthrough  SumFdbkVariant=Disabled  SumVariant=Sum_PID
  PS-Simulink Converter : nesl_utility/PS-Simulink Converter  PhysicalDomain=network_engine_domain  SubClassName=ps_output  LeftPortType=input  RightPortType=output  PseudoPeriodic=off  Frequencies=[]  Unit=rad  AffineConversion=off
  Sum : Sum  Inputs=|+-
  q : PMIOPort  Side=Left
  t : Outport
  wires:
  PID Controller/1 -> t/1
  Sum/1 -> PID Controller/1
  PS-Simulink Converter/1 -> Memory/1
  qref/1 -> Sum/1
  Memory/1 -> Sum/2
  connections:
  q/RConn1 -- PS-Simulink Converter/LConn1

== system Biped_Model/Robot/Robot Leg L/Knee Joint/Motor/Joint Servo ==
  qref : Inport
  Abs : Abs
  Controlled Voltage Source : fl_lib/Electrical/Electrical Sources/Controlled Voltage Source
  Controlled Voltage Source1 : fl_lib/Electrical/Electrical Sources/Controlled Voltage Source
  Electrical Reference : fl_lib/Electrical/Electrical Elements/Electrical Reference
  PID Controller : simulink/Continuous/PID Controller  Controller=PID  Form=Parallel  TimeDomain=Continuous-time  SampleTime=-1  IntegratorMethod=Forward Euler  FilterMethod=Forward Euler  ControllerParametersSource=internal  P=Kp  I=Ki  D=Kd  UseFilter=on  N=N  TunerSelectOption=Transfer Function Based (PID Tuner App)  ZeroCross=off  InitialConditionSource=internal  InitialConditionForIntegrator=0  InitialConditionForFilter=0  DifferentiatorICPrevScaledInput=0  ExternalReset=none  TrackingMode=off  Kt=1  LimitOutput=on  UpperSaturationLimit=Tmax  LowerSaturationLimit=-Tmax  LinearizeAsGain=on  AntiWindupMode=clamping  Kb=1  POutMin=[]  POutMax=[]  IOutMin=[]  IOutMax=[]  DOutMin=[]  DOutMax=[]  NOutMin=[]  NOutMax=[]  SumOutMin=[]  SumOutMax=[]  SaturationOutMin=[]  SaturationOutMax=[]  PParamMin=[]  PParamMax=[]  IParamMin=[]  IParamMax=[]  DParamMin=[]  DParamMax=[]  NParamMin=[]  NParamMax=[]  KbParamMin=[]  KbParamMax=[]  KtParamMin=[]  KtParamMax=[]  KbOutMin=[]  KbOutMax=[]  KtOutMin=[]  KtOutMax=[]  IntegratorOutMin=[]  IntegratorOutMax=[]  FilterOutMin=[]  FilterOutMax=[]  SumI1OutMin=[]  SumI1OutMax=[]  SumI2OutMin=[]  SumI2OutMax=[]  SumI3OutMin=[]  SumI3OutMax=[]  SumI4OutMin=[]  SumI4OutMax=[]  SumDOutMin=[]  SumDOutMax=[]  DifferentiatorOutMin=[]  DifferentiatorOutMax=[]  FilterDiffOutCoefMin=[]  FilterDiffOutCoefMax=[]  ReciprocalOutMin=[]  ReciprocalOutMax=[]  SumDenOutMin=[]  SumDenOutMax=[]  SumNumOutMin=[]  SumNumOutMax=[]  DivideOutMin=[]  DivideOutMax=[]  IntegratorContinuousStateAttributes=''  IntegratorStateMustResolveToSignalObject=off  IntegratorRTWStateStorageClass=Auto  FilterContinuousStateAttributes=''  FilterStateMustResolveToSignalObject=off  FilterRTWStateStorageClass=Auto  ParallelPVariant=InternalParameters  IdealPVariant=Disabled  IVariant=InternalParameters  DVariant=InternalParameters  IntegratorVariant=Continuous  SatVariant=Enabled  AWVariant=ContClampingParallel  PCopyVariant=Disabled  TRVariant=Disabled  FdbkBlocksVariant=Forward  IdealPFdbkVariant=Disabled  SatFdbkVariant=Disabled  DerivativeFilterVariant=ContFilter  NVariant=InternalParameters  NCopyVariant=Disabled  FilterICVariant=InternalICsFilter  IntegratorICVariant=InternalICs  ExternalResetVariant=Disabled  TRSumVariant=Passthrough  SumFdbkVariant=Disabled  SumVariant=Sum_PID
  PS-Simulink Converter : nesl_utility/PS-Simulink Converter  PhysicalDomain=network_engine_domain  SubClassName=ps_output  LeftPortType=input  RightPortType=output  PseudoPeriodic=off  Frequencies=[]  Unit=rad  AffineConversion=off
  Relay : Relay  OnSwitchValue=1e-3  OffSwitchValue=-1e-3  OnOutputValue=0  OffOutputValue=5
  Simulink-PS Converter : nesl_utility/Simulink-PS Converter  PhysicalDomain=network_engine_domain  SubClassName=ps_input  LeftPortType=input  RightPortType=output  PseudoPeriodic=off  Frequencies=[]  NoiseDistribution=none  NoiseParameters=[]  Unit=1  AffineConversion=off  FilteringAndDerivatives=provide  SimscapeFilterOrder=1  InputFilterTimeConstant=0.005  UdotUserProvided=0
  Simulink-PS Converter1 : nesl_utility/Simulink-PS Converter  PhysicalDomain=network_engine_domain  SubClassName=ps_input  LeftPortType=input  RightPortType=output  PseudoPeriodic=off  Frequencies=[]  NoiseDistribution=none  NoiseParameters=[]  Unit=1  AffineConversion=off  FilteringAndDerivatives=provide  SimscapeFilterOrder=1  InputFilterTimeConstant=0.005  UdotUserProvided=0
  Sum : Sum  Inputs=|+-
  q : PMIOPort  Side=Left
  V : PMIOPort  Port=2  Side=Right
  REV : PMIOPort  Port=3  Side=Right
  wires:
  PID Controller/1 -> Abs/1, Relay/1
  qref/1 -> Sum/1
  PS-Simulink Converter/1 -> Sum/2
  Sum/1 -> PID Controller/1
  Abs/1 -> Simulink-PS Converter/1
  Relay/1 -> Simulink-PS Converter1/1
  connections:
  q/RConn1 -- PS-Simulink Converter/LConn1
  Simulink-PS Converter/RConn1 -- Controlled Voltage Source/RConn1
  Controlled Voltage Source/LConn1 -- V/RConn1
  Electrical Reference/LConn1 -- Controlled Voltage Source/RConn2 -- Controlled Voltage Source1/RConn2
  Controlled Voltage Source1/LConn1 -- REV/RConn1
  Simulink-PS Converter1/RConn1 -- Controlled Voltage Source1/RConn1

== system Biped_Model/Robot/Robot Leg L/Knee Joint/Torque/Joint Servo ==
  qref : Inport
  Memory : Memory
  PID Controller : simulink/Continuous/PID Controller  Controller=PID  Form=Parallel  TimeDomain=Continuous-time  SampleTime=-1  IntegratorMethod=Forward Euler  FilterMethod=Forward Euler  ControllerParametersSource=internal  P=Kp  I=Ki  D=Kd  UseFilter=on  N=N  TunerSelectOption=Transfer Function Based (PID Tuner App)  ZeroCross=off  InitialConditionSource=internal  InitialConditionForIntegrator=0  InitialConditionForFilter=0  DifferentiatorICPrevScaledInput=0  ExternalReset=none  TrackingMode=off  Kt=1  LimitOutput=on  UpperSaturationLimit=Tmax  LowerSaturationLimit=-Tmax  LinearizeAsGain=on  AntiWindupMode=clamping  Kb=1  POutMin=[]  POutMax=[]  IOutMin=[]  IOutMax=[]  DOutMin=[]  DOutMax=[]  NOutMin=[]  NOutMax=[]  SumOutMin=[]  SumOutMax=[]  SaturationOutMin=[]  SaturationOutMax=[]  PParamMin=[]  PParamMax=[]  IParamMin=[]  IParamMax=[]  DParamMin=[]  DParamMax=[]  NParamMin=[]  NParamMax=[]  KbParamMin=[]  KbParamMax=[]  KtParamMin=[]  KtParamMax=[]  KbOutMin=[]  KbOutMax=[]  KtOutMin=[]  KtOutMax=[]  IntegratorOutMin=[]  IntegratorOutMax=[]  FilterOutMin=[]  FilterOutMax=[]  SumI1OutMin=[]  SumI1OutMax=[]  SumI2OutMin=[]  SumI2OutMax=[]  SumI3OutMin=[]  SumI3OutMax=[]  SumI4OutMin=[]  SumI4OutMax=[]  SumDOutMin=[]  SumDOutMax=[]  DifferentiatorOutMin=[]  DifferentiatorOutMax=[]  FilterDiffOutCoefMin=[]  FilterDiffOutCoefMax=[]  ReciprocalOutMin=[]  ReciprocalOutMax=[]  SumDenOutMin=[]  SumDenOutMax=[]  SumNumOutMin=[]  SumNumOutMax=[]  DivideOutMin=[]  DivideOutMax=[]  IntegratorContinuousStateAttributes=''  IntegratorStateMustResolveToSignalObject=off  IntegratorRTWStateStorageClass=Auto  FilterContinuousStateAttributes=''  FilterStateMustResolveToSignalObject=off  FilterRTWStateStorageClass=Auto  ParallelPVariant=InternalParameters  IdealPVariant=Disabled  IVariant=InternalParameters  DVariant=InternalParameters  IntegratorVariant=Continuous  SatVariant=Enabled  AWVariant=ContClampingParallel  PCopyVariant=Disabled  TRVariant=Disabled  FdbkBlocksVariant=Forward  IdealPFdbkVariant=Disabled  SatFdbkVariant=Disabled  DerivativeFilterVariant=ContFilter  NVariant=InternalParameters  NCopyVariant=Disabled  FilterICVariant=InternalICsFilter  IntegratorICVariant=InternalICs  ExternalResetVariant=Disabled  TRSumVariant=Passthrough  SumFdbkVariant=Disabled  SumVariant=Sum_PID
  PS-Simulink Converter : nesl_utility/PS-Simulink Converter  PhysicalDomain=network_engine_domain  SubClassName=ps_output  LeftPortType=input  RightPortType=output  PseudoPeriodic=off  Frequencies=[]  Unit=rad  AffineConversion=off
  Sum : Sum  Inputs=|+-
  q : PMIOPort  Side=Left
  t : Outport
  wires:
  PID Controller/1 -> t/1
  Sum/1 -> PID Controller/1
  PS-Simulink Converter/1 -> Memory/1
  qref/1 -> Sum/1
  Memory/1 -> Sum/2
  connections:
  q/RConn1 -- PS-Simulink Converter/LConn1
